simulink model "Task_4"  (R2015a)
settings: Solver=ode45  StartTime=0.0  StopTime=10.0  RelTol=1e-3
settings Model: Creator=acer  LastModifiedBy=acer

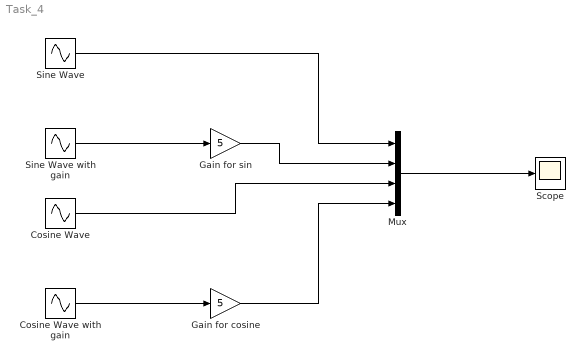
== system Task_4 ==
  Cosine Wave : Sin  Phase=pi/2  SampleTime=0
  Cosine Wave with gain : Sin  Phase=pi/2  SampleTime=0
  Gain for cosine : Gain  Gain=5
  Gain for sin : Gain  Gain=5
  Mux : Mux
  Scope : Scope
      settings: ShowLegends=on
  Sine Wave : Sin  SampleTime=0
  Sine Wave with gain : Sin  SampleTime=0
  wires:
  Mux/1 -> Scope/1
  Sine Wave/1 -> Mux/1
  Sine Wave with gain/1 -> Gain for sin/1
  Gain for sin/1 -> Mux/2
  Cosine Wave/1 -> Mux/3
  Cosine Wave with gain/1 -> Gain for cosine/1
  Gain for cosine/1 -> Mux/4
